simulink library "Window_with_Shading"  (Simulink 8.2)
settings: Solver=ode45  StartTime=0.0  StopTime=10.0  RelTol=1e-3
libraries: carnot x1
settings Model: Creator=lena.frank  LastModifiedBy=drhf

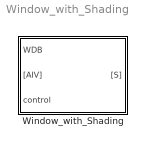
== system Window_with_Shading ==
  Window_with_Shading : Subsystem  mask(window){windowsize=[1 1], numpanes=2, frame=0.15, pos=0, d=[0.004 0.004], rho=[2500 2500], cp=[0.21 0.21]*3600, t0=20, misc=[0.2 0.1 0.84 0.84], gvalue=0.6, tauzero=0.58, Ug=1.4, shad_type=No shading, type_glazing=Dreifach-Wärmeschutzglas, tau_shad=0.304, bli_a=0.08, bli_b=0.0126, bli_c=0.009, bli_d=0.062, bli_alpha=45, bli_refl=0.441}
      mask prompts: windowsize "size of window [m] [height width]"; numpanes "number of window panes [1..4]"; frame "part of frame of the surface (0..1)"; pos "azimut (0=south, east = -90)"; d "thickness of panes [m]"; rho "density of glass [kg/m³]"; cp "capacity of glass [J/(kgK)]"; t0 "initial temperature [degree centigrade]"; misc "[reflection_ground absorption_out emission_out emission_in]"; gvalue "energy transmission of window (g-value) [0..1]"; tauzero "transmission of glass [0..1]"; Ug "heat transfer coefficient (U-value) [W/m²K]"; shad_type "shading type [no Shading/exterior/interior]"; type_glazing "glazing type"; tau_shad "solar transmittance of shading element [0..1]"; bli_a "a  Depth of blind blades [m]"; bli_b "b heigth of blind blades [m]"; bli_c "c distance of "b" to back end of blind blade [m]"; bli_d "d offset between blind blades [m]"; bli_alpha "blind angle  (0=closed, 90=horizontal) [0..90]"; bli_refl "optical reflectance of blind surface [0..1]"
      mask help:
      | The window model evaluates the g-value, the total energy transmission tau and the u-value to build up a two node model.
      |
      | control [0..1]:   specifies the fraction of the shading device.
      |                   0 means a norm g-value, 1 means total shading of the
      |                   window
      mask init:
      | pos = [90  pos  0];
      | 
      | h = windowsize(1);
      | w = windowsize(2);
      | 
      | %für Variablen in surfrad
      | reflectground = max(0, min(1, misc(1)));
      | 
      | %windowangle = position(1);
      | %windowazimut = position(2);
      | %windowheight=h;
      | %windowwidth=w;
      | windowsurface = h*w;
      | 
      | absorption_out = misc(2);
      | emission_out = misc(3);
      | emission_in = misc(4);
      | 
      | for i = 1:numpanes
      | C = sum(cp(i)*d(i)*d(i)*rho(i));
      | end
      | R=1/Ug-(0.04+0.13);
      | timeconst = R*C/2;
      | 
      | R_norm_in = 0.13;
      | R_norm_out = 0.04;
      | Rwin = 1/Ug - R_norm_in - R_norm_out;
      mask Help: web(fullfile(path_carnot('help'),'Window.html'),'-helpbrowser')
      mask TypeOptions shad_type: No shading | Exterior Screen | Interior Screen | Venetian Blind
      mask Callback shad_type:
      | switch get_param(gcb,'shad_type')
      |         case 'No shading' % nr. 1 no shading
      |             set_param(gcb,'MaskVisibilities',{'on','on','on','on','on','on','on','on','on','on','on','on','on','off','off','off','off','off','off','off','off'});
      |         case 'Exterior Screen' % nr. 2 external screen
      |             set_param(gcb,'MaskVisibilities',{'on','on','on','on','on','on','on','on','on','on','on','on','on','off','on','off','off','off','off','off','off'});
      |         case 'Interior Screen' % nr. 3 Interior Screen
      |             set_param(gcb,'MaskVisibilities',{'on','on','on','on','on','on','on','on','on','on','on','on','on','on','on','off','off','off','off','off','off'});
      |         case 'Venetian Blind' % nr. 4 venetian blind
      |             set_param(gcb,'MaskVisibilities',{'on','on','on','on','on','on','on','on','on','on','on','on','on','off','off','on','on','on','on','on','on'});
      |     end
      mask TypeOptions type_glazing: Zweifachglas normal | Zweifach-Wärmeschutzglas | Zweifach-Kombiglas 73/41 | Zweifach-Kombiglas 50/24 | Dreifachglas normal | Dreifach-Wärmeschutzglas

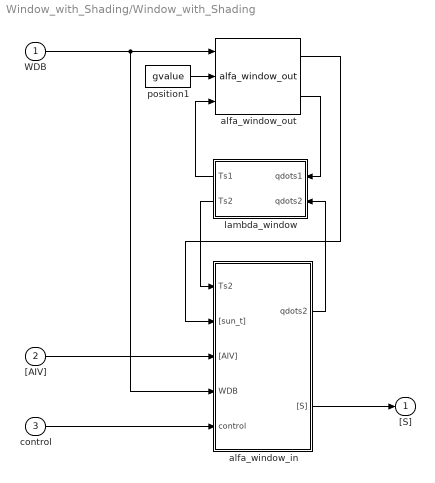
== system Window_with_Shading/Window_with_Shading ==
  WDB : Inport
  "[AIV]" : Inport  Port=2
  control : Inport  Port=3
  alfa_window_in : Subsystem  mask(ALFA){}
      mask help:
      | Convective and radiative heat transfer at the INDOOR SURFACE OF A VERTICAL WINDOW with 1-4 layers (each 3 ... 8 mm thick).
      |
      | Ts  : temperature of window surface, °C,
      | [sun_t]  : sun data (incidence angle, direct and diffuse radiation
      |     at tilted window surface),
      | [AIV]  : conditions of zone node,
      | qdots  : specific heat flow into window construction, W/m^2,
      | [S]  : heat and air flow to zone node.
  alfa_window_out : carnot/Load/Houses/heat_transfer/alfa_window_out
  lambda_window : Subsystem  mask(LAMBDA){}
      mask help:
      | Heat conduction through a transparent component (window).
      |
      | qdots1	: specific heat flow vertical on surface 1, W/m²
      | qdots2	: specific heat flow vertical on surface 2, W/m²
      | Ts1	: temperature of surface 1, °C
      | Ts2	: temperature of surface 2, °C
      |
      | NOTE CONVENTION for INPUT NUMBER:
      | "1"	  indoor surface of an outer window OR
      | 	  surface "a" of an inner window OR
      |  	  surface "f" of a glass floor
      |
      | "2"	  outdoor surface of a window OR
      | 	  surface "b" of an inner window OR
      |  	  surface "c" of a glass ceiling
  position1 : Constant  Value=gvalue
  "[S]" : Outport
  wires:
  position1/1 -> alfa_window_out/2
  control/1 -> alfa_window_in/5(control)
  alfa_window_out/1 -> alfa_window_in/2("[sun_t]")
  alfa_window_out/2 -> lambda_window/1(qdots1)
  lambda_window/2(Ts2) -> alfa_window_in/1(Ts2)
  alfa_window_in/2("[S]") -> "[S]"/1
  alfa_window_in/1(qdots2) -> lambda_window/2(qdots2)
  "[AIV]"/1 -> alfa_window_in/3("[AIV]")
  WDB/1 -> alfa_window_out/1, alfa_window_in/4(WDB)
  lambda_window/1(Ts1) -> alfa_window_out/3

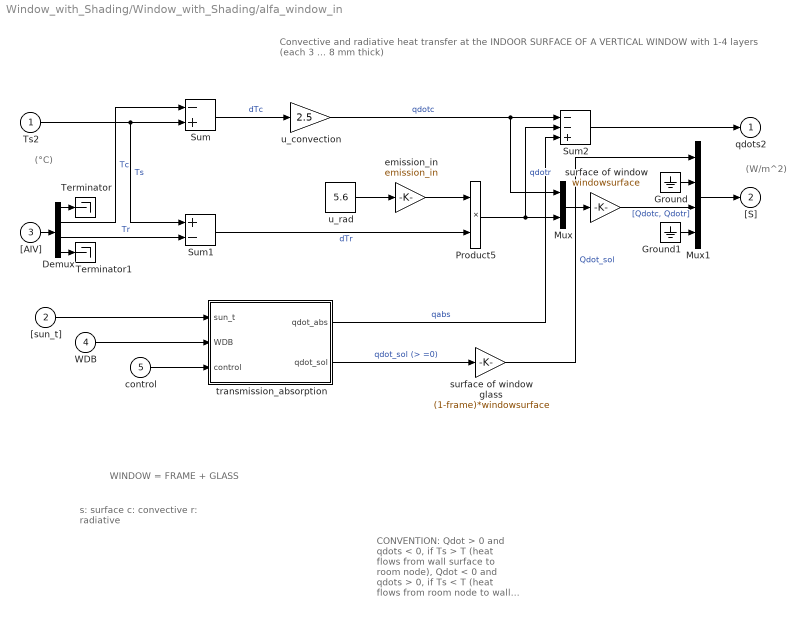
== system Window_with_Shading/Window_with_Shading/alfa_window_in ==
  note: (°C)
  note: Convective and radiative heat transfer at the INDOOR SURFACE OF A VERTICAL WINDOW
      | with 1-4 layers (each 3 ... 8 mm thick)
  note: WINDOW = FRAME + GLASS
  note: s: surface
      | c: convective
      | r: radiative
  note: CONVENTION:
      | Qdot > 0 and qdots < 0, if Ts > T (heat flows from wall surface to room node),
      | Qdot < 0 and qdots > 0, if Ts < T (heat flows from room node to wall surface).
  note: (W/m^2)
  Ts2 : Inport
  "[sun_t]" : Inport  Port=2
  "[AIV]" : Inport  Port=3
  WDB : Inport  Port=4
  control : Inport  Port=5
  Demux : Demux  Outputs=[1 1 1 6]
  Ground : Ground
  Ground1 : Ground
  Mux : Mux  Inputs=2
  Mux1 : Mux  Inputs=[1 5 2 5]
  Product5 : Product  SaturateOnIntegerOverflow=on  RndMeth=Zero  InputSameDT=on  OutDataTypeStr=Inherit: Same as first input
  Sum : Sum  Inputs=-+  SaturateOnIntegerOverflow=on  InputSameDT=on  OutDataTypeStr=Inherit: Same as first input
  Sum1 : Sum  Inputs=+-  SaturateOnIntegerOverflow=on  InputSameDT=on  OutDataTypeStr=Inherit: Same as first input
  Sum2 : Sum  Inputs=--+  SaturateOnIntegerOverflow=on  InputSameDT=on  OutDataTypeStr=Inherit: Same as first input
  Terminator : Terminator
  Terminator1 : Terminator
  emission_in : Gain  Gain=emission_in  SaturateOnIntegerOverflow=on  OutDataTypeStr=Inherit: Same as input  ParamDataTypeStr=Inherit: Same as input
  surface of window : Gain  Gain=windowsurface  SaturateOnIntegerOverflow=on  OutDataTypeStr=Inherit: Same as input  ParamDataTypeStr=Inherit: Same as input
  surface of window glass : Gain  Gain=(1-frame)*windowsurface  SaturateOnIntegerOverflow=on  OutDataTypeStr=Inherit: Same as input  ParamDataTypeStr=Inherit: Same as input
  transmission_absorption : Subsystem
  u_convection : Gain  Gain=2.5  SaturateOnIntegerOverflow=on  OutDataTypeStr=Inherit: Same as input  ParamDataTypeStr=Inherit: Same as input
  u_rad : Constant  Value=5.6
  qdots2 : Outport
  "[S]" : Outport  Port=2
  wires:
  control/1 -> transmission_absorption/3(control)
  WDB/1 -> transmission_absorption/2(WDB)
  transmission_absorption/1(qdot_abs) -> Sum2/3  "qabs"
  transmission_absorption/2(qdot_sol) -> surface of window glass/1  "qdot_sol (> =0)"
  Demux/3 -> Sum1/2  "Tr"
  Sum/1 -> u_convection/1  "dTc"
  Demux/2 -> Sum/1  "Tc"
  surface of window/1 -> Mux1/3  "[Qdotc, Qdotr]"
  surface of window glass/1 -> Mux1/1  "Qdot_sol"
  "[sun_t]"/1 -> transmission_absorption/1(sun_t)
  u_convection/1 -> Mux/1, Sum2/1  "qdotc"
  Product5/1 -> Sum2/2, Mux/2  "qdotr"
  Ts2/1 -> Sum1/1, Sum/2  "Ts"
  u_rad/1 -> emission_in/1
  Sum1/1 -> Product5/2  "dTr"
  emission_in/1 -> Product5/1
  Mux/1 -> surface of window/1
  Demux/1 -> Terminator/1
  "[AIV]"/1 -> Demux/1
  Demux/4 -> Terminator1/1
  Sum2/1 -> qdots2/1
  Mux1/1 -> "[S]"/1
  Ground/1 -> Mux1/2
  Ground1/1 -> Mux1/4

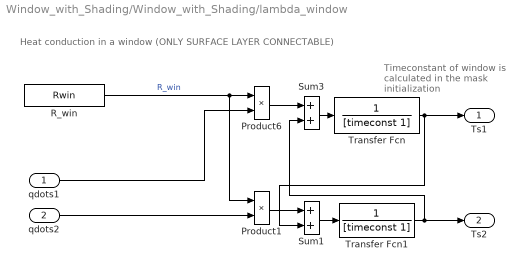
== system Window_with_Shading/Window_with_Shading/lambda_window ==
  note: Heat conduction in a window (ONLY SURFACE LAYER CONNECTABLE)
  note: Timeconstant of window is calculated
      | in the mask initialization
  qdots1 : Inport
  qdots2 : Inport  Port=2
  Product1 : Product  SaturateOnIntegerOverflow=on  RndMeth=Zero  InputSameDT=on  OutDataTypeStr=Inherit: Same as first input
  Product6 : Product  SaturateOnIntegerOverflow=on  RndMeth=Zero  InputSameDT=on  OutDataTypeStr=Inherit: Same as first input
  R_win : Constant  Value=Rwin
  Sum1 : Sum  SaturateOnIntegerOverflow=on  InputSameDT=on  OutDataTypeStr=Inherit: Same as first input
  Sum3 : Sum  SaturateOnIntegerOverflow=on  InputSameDT=on  OutDataTypeStr=Inherit: Same as first input
  Transfer Fcn : TransferFcn  Denominator=[timeconst 1]
  Transfer Fcn1 : TransferFcn  Denominator=[timeconst 1]
  Ts1 : Outport
  Ts2 : Outport  Port=2
  wires:
  Transfer Fcn1/1 -> Ts2/1, Sum3/2
  Transfer Fcn/1 -> Ts1/1, Sum1/2
  qdots1/1 -> Product6/2
  qdots2/1 -> Product1/2
  Product6/1 -> Sum3/1
  Sum3/1 -> Transfer Fcn/1
  Product1/1 -> Sum1/1
  Sum1/1 -> Transfer Fcn1/1
  R_win/1 -> Product6/1, Product1/1  "R_win"

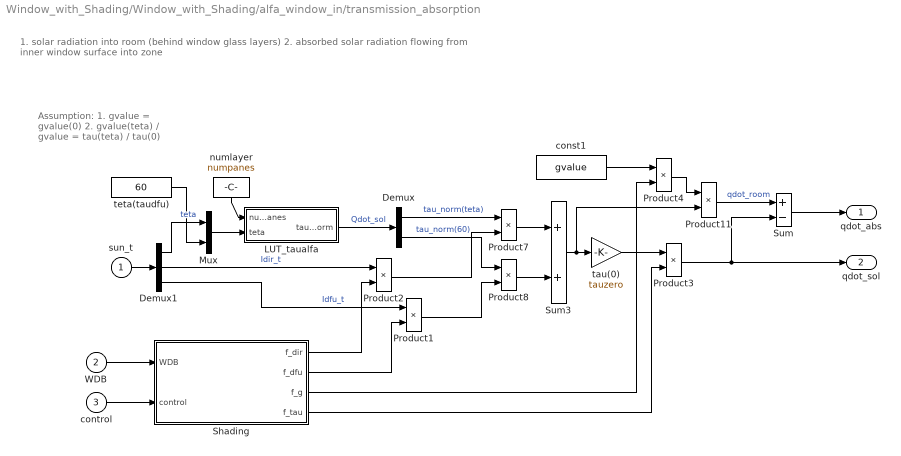
== system Window_with_Shading/Window_with_Shading/alfa_window_in/transmission_absorption ==
  note: Assumption:
      | 1. gvalue = gvalue(0)
      | 2. gvalue(teta) / gvalue = tau(teta) / tau(0)
  note: 1. solar radiation into room (behind window glass layers)
      | 2. absorbed solar radiation flowing from inner window surface into zone
  sun_t : Inport
  WDB : Inport  Port=2
  control : Inport  Port=3
  Demux : Demux  Outputs=2
  Demux1 : Demux  Outputs=3
  LUT_taualfa : Subsystem  mask(LOOK UP TABLE){}
      mask help:
      | Normalized RADIATION TRANSMISSION COEFFICIENT of a window glass layer stack with 1, 2, 3 or 4 layers depending on the incidence angle.
      |
      | teta		: incidence angle = angle between surface normal and
      | 	                incidence direction, degree
      | numlayer	: number of layers within the window glass, [1,4].
      | tau		: transmission of glass layer stack, [0,1]
      |
      | NOTE: This block is defined for pane thickness between 3 and 6 mm.
  Mux : Mux  Inputs=2
  Product{1..4,7..8} (6 alike) : Product  SaturateOnIntegerOverflow=on  RndMeth=Zero  InputSameDT=on  OutDataTypeStr=Inherit: Same as first input
  Product11 : Product  Inputs=**  SaturateOnIntegerOverflow=on  RndMeth=Zero  InputSameDT=on  OutDataTypeStr=Inherit: Same as first input
  Shading : Subsystem
  Sum : Sum  Inputs=+-  SaturateOnIntegerOverflow=on  InputSameDT=on  OutDataTypeStr=Inherit: Same as first input
  Sum3 : Sum  SaturateOnIntegerOverflow=on  InputSameDT=on  OutDataTypeStr=Inherit: Same as first input
  const1 : Constant  Value=gvalue
  numlayer : Constant  Value=numpanes
  tau(0) : Gain  Gain=tauzero  SaturateOnIntegerOverflow=on  OutDataTypeStr=Inherit: Same as input  ParamDataTypeStr=Inherit: Same as input
  teta(taudfu) : Constant  Value=60
  qdot_abs : Outport
  qdot_sol : Outport  Port=2
  wires:
  control/1 -> Shading/2(control)
  WDB/1 -> Shading/1(WDB)
  Shading/3(f_g) -> Product4/2
  const1/1 -> Product4/1
  Product4/1 -> Product11/1
  Shading/4(f_tau) -> Product3/2
  Shading/2(f_dfu) -> Product1/2
  Shading/1(f_dir) -> Product2/2
  Product2/1 -> Product7/2
  Demux1/2 -> Product2/1  "Idir_t"
  Product1/1 -> Product8/2
  Demux1/3 -> Product1/1  "Idfu_t"
  Product3/1 -> qdot_sol/1, Sum/2
  tau(0)/1 -> Product3/1
  sun_t/1 -> Demux1/1
  LUT_taualfa/1(tau_norm) -> Demux/1  "Qdot_sol"
  Demux/1 -> Product7/1  "tau_norm(teta)"
  Product7/1 -> Sum3/1
  Product8/1 -> Sum3/2
  Sum3/1 -> Product11/2, tau(0)/1
  Demux/2 -> Product8/1  "tau_norm(60)"
  Product11/1 -> Sum/1  "qdot_room"
  Sum/1 -> qdot_abs/1
  Demux1/1 -> Mux/1  "teta"
  teta(taudfu)/1 -> Mux/2
  numlayer/1 -> LUT_taualfa/1(numlpanes)
  Mux/1 -> LUT_taualfa/2(teta)

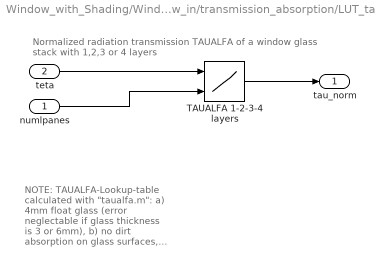
== system Window_with_Shading/Window_with_Shading/alfa_window_in/transmission_absorption/LUT_taualfa ==
  note: NOTE:
      | TAUALFA-Lookup-table calculated with "taualfa.m":
      |   a) 4mm float glass (error neglectable if glass thickness is 3 or 6mm),
      |   b) no dirt absorption on glass surfaces,
      |   c) 100% room absorption,
      |   d) normalized to tau(0).
      |
      | From: Duffie / Beckman: Solar Engineering of Thermal Processes, 1991
  note: Normalized radiation transmission TAUALFA
      | of a window glass stack with 1,2,3 or 4 layers
  numlpanes : Inport
  teta : Inport  Port=2
  TAUALFA 1-2-3-4 layers : Lookup2D  RowIndex=[0:10:90]  ColumnIndex=[1:4]  Table="[1  1  1  1;.99955 .99912  .9987 .99827;.99787  .9961 .99449 .99298;.99364 .98941 .98618 .98366;.98364 .97519 .97041 .96824;.9601 .94337 .93638 .93624;.90423 .86634 .84734 .84064;.77129 .67843 .61507 .56891;.47436  .3235 .22952 .16682;0  0  0  0]"  SaturateOnIntegerOverflow=on  InputSameDT=on
  tau_norm : Outport
  wires:
  teta/1 -> TAUALFA 1-2-3-4 layers/1
  numlpanes/1 -> TAUALFA 1-2-3-4 layers/2
  TAUALFA 1-2-3-4 layers/1 -> tau_norm/1

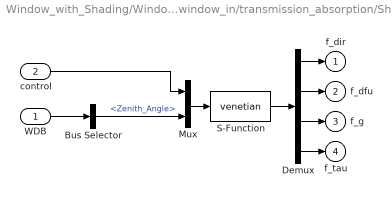
== system Window_with_Shading/Window_with_Shading/alfa_window_in/transmission_absorption/Shading ==
  WDB : Inport
  control : Inport  Port=2
  Bus Selector : BusSelector  OutputSignals=Zenith_Angle
  Demux : Demux
  Mux : Mux  Inputs=2
  S-Function : S-Function  FunctionName=venetian  Parameters=bli_a, bli_b, bli_c, bli_d, bli_alpha, bli_refl, shad_type, type_glazing, tau_shad  EnableBusSupport=off
  f_dir : Outport
  f_dfu : Outport  Port=2
  f_g : Outport  Port=3
  f_tau : Outport  Port=4
  wires:
  WDB/1 -> Bus Selector/1
  Bus Selector/1 -> Mux/2  "<Zenith_Angle>"
  control/1 -> Mux/1
  Mux/1 -> S-Function/1
  S-Function/1 -> Demux/1
  Demux/1 -> f_dir/1
  Demux/2 -> f_dfu/1
  Demux/3 -> f_g/1
  Demux/4 -> f_tau/1
